simulink model "bicycle_kin_planCont"  (R2020b)
settings: Solver=FixedStepAuto  StartTime=0.0  StopTime=inf  FixedStep=0.02  RelTol=1e-3
model workspace (MAT data in the model file):
  SL_ROS_VariableLengthArrays_MaxSizes.CommonInfo.ArrayTruncateAction = 'EmitWarning'
  SL_ROS_VariableLengthArrays_MaxSizes.MsgTypeMap = containers.Map
  SL_ROS_VariableLengthArrays_MaxSizes.MsgTypeMap.serialization.keys = {'nav_msgs/Path'}
  SL_ROS_VariableLengthArrays_MaxSizes.MsgTypeMap.serialization.values{1}.PropertyName = 'Poses'
  SL_ROS_VariableLengthArrays_MaxSizes.MsgTypeMap.serialization.values{1}.DataType = 'geometry_msgs/PoseStamped'
  SL_ROS_VariableLengthArrays_MaxSizes.MsgTypeMap.serialization.values{1}.MaxLength = 25
  SL_ROS_VariableLengthArrays_MaxSizes.MsgTypeMap.serialization.uniformity = 0
  SL_ROS_VariableLengthArrays_MaxSizes.MsgTypeMap.serialization.keyType = 'char'
  SL_ROS_VariableLengthArrays_MaxSizes.MsgTypeMap.serialization.valueType = 'any'
undefined symbols (not defined in the file or in its folder): Angular, Linear
libraries: robotlib x12
settings Model: Creator=bascetta  LastModifiedBy=root
settings OptimizationCC: EnhancedBackFolding=on  PassReuseOutputArgsAs=Individual arguments  ZeroExternalMemoryAtStartup=off  ZeroInternalMemoryAtStartup=off  MaxStackSize=64  OptimizeBlockOrder=speed  DifferentSizesBufferReuse=on  OptimizationCustomize=off  EfficientTunableParamExpr=on
settings DebuggingCC: ParameterTunabilityLossMsg=error
settings HardwareCC: ProdBitPerPointer=32  ProdBitPerSizeT=32  ProdBitPerPtrDiffT=32  ProdLargestAtomicFloat=None  ProdIntDivRoundTo=Undefined  ProdEndianess=Unspecified  ProdWordSize=32  ProdHWDeviceType=Generic->Unspecified (assume 32-bit Generic)
settings SFSimCC: MATLABDynamicMemAlloc=off  SimTargetLang=C++
settings RTWCC: Description=Embedded Coder  SystemTargetFile=ert.tlc  HardwareBoard=Robot Operating System (ROS)  TLCOptions="-aInlineSetEventsForThisBaseRateFcn=TLC_FALSE -aSuppressMultiTaskScheduler=TLC_FALSE  -aRateBasedStepFcn=0"  GenCodeOnly=on  TemplateMakefile=ert_default_tmf  Toolchain=Catkin  TargetLang=C++
settings CodeAppCC: ForceParamTrailComments=on  IgnoreCustomStorageClasses=off  OperatorAnnotations=on  SimulinkDataObjDesc=on  SFDataObjDesc=on  InsertBlockDesc=on
settings ERTTargetCC: SupportVariableSizeSignals=on  ERTCustomFileTemplate=rostime_codertarget_file_process.tlc

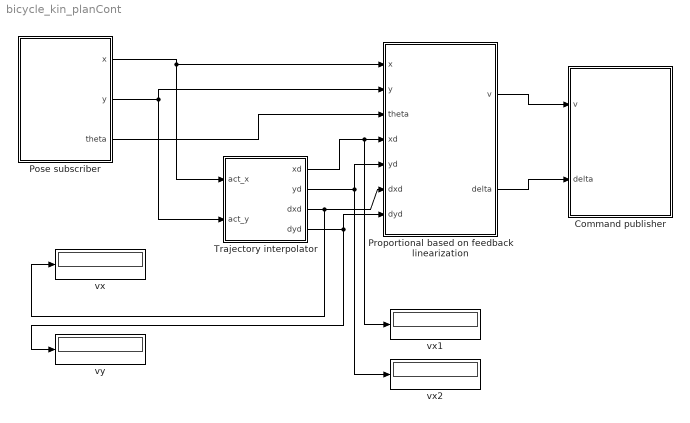
== system bicycle_kin_planCont ==
  Command publisher : Subsystem  mask{simPublishRate=50}
      mask prompts: simPublishRate "Publising rate [Hz]"
  Pose subscriber : Subsystem
  Proportional based on feedback linearization : Subsystem  mask{KP=0.5, Epsilon=0.5}
      mask prompts: KP "Proportional gain"; Epsilon "Distance of the point"
      mask TypeOptions Epsilon: point distance/Value
  Trajectory interpolator : Subsystem  mask{R=2.0}
      mask prompts: R "Ball radius to switch from one point to another"
  vx : Display
  vx1 : Display
  vx2 : Display
  vy : Display
  wires:
  Proportional based on feedback linearization/1(v) -> Command publisher/1(v)
  Proportional based on feedback linearization/2(delta) -> Command publisher/2(delta)
  Pose subscriber/1(x) -> Trajectory interpolator/1(act_x), Proportional based on feedback linearization/1(x)
  Pose subscriber/2(y) -> Trajectory interpolator/2(act_y), Proportional based on feedback linearization/2(y)
  Pose subscriber/3(theta) -> Proportional based on feedback linearization/3(theta)
  Trajectory interpolator/1(xd) -> Proportional based on feedback linearization/4(xd), vx1/1
  Trajectory interpolator/2(yd) -> vx2/1, Proportional based on feedback linearization/5(yd)
  Trajectory interpolator/3(dxd) -> vx/1, Proportional based on feedback linearization/6(dxd)
  Trajectory interpolator/4(dyd) -> vy/1, Proportional based on feedback linearization/7(dyd)

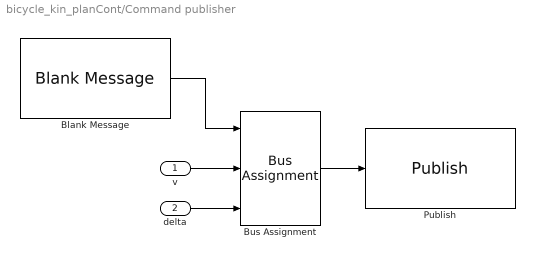
== system bicycle_kin_planCont/Command publisher ==
  v : Inport  SampleTime=1/simPublishRate
  delta : Inport  Port=2  SampleTime=1/simPublishRate
  Blank Message : robotlib/Blank Message  messageClass=Message  entityType=geometry_msgs/Twist  messageType=geometry_msgs/Twist  SampleTime=1/simPublishRate  legacyBusStruct=off
  Bus Assignment : BusAssignment  AssignedSignals=Linear.X,Angular.Z
  Publish : robotlib/Publish  topicSource=Specify your own  topic=/cmd_vel  messageType=geometry_msgs/Twist  legacyBusStruct=off  messageQueueLength=1
  wires:
  Bus Assignment/1 -> Publish/1
  Blank Message/1 -> Bus Assignment/1
  v/1 -> Bus Assignment/2
  delta/1 -> Bus Assignment/3

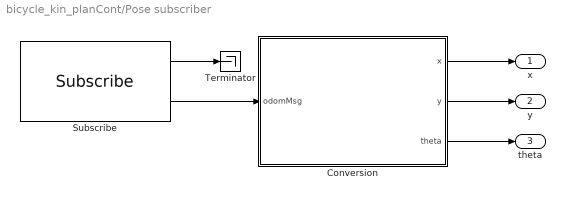
== system bicycle_kin_planCont/Pose subscriber ==
  Conversion : MATLAB Function  TreatAsAtomicUnit=on
  Subscribe : robotlib/Subscribe  topicSource=Specify your own  topic=/odom  messageType=nav_msgs/Odometry  SampleTime=-1  legacyBusStruct=off  messageQueueLength=1
  Terminator : Terminator
  x : Outport
  y : Outport  Port=2
  theta : Outport  Port=3
  wires:
  Subscribe/1 -> Terminator/1
  Subscribe/2 -> Conversion/1(odomMsg)
  Conversion/1(x) -> x/1
  Conversion/2(y) -> y/1
  Conversion/3(theta) -> theta/1

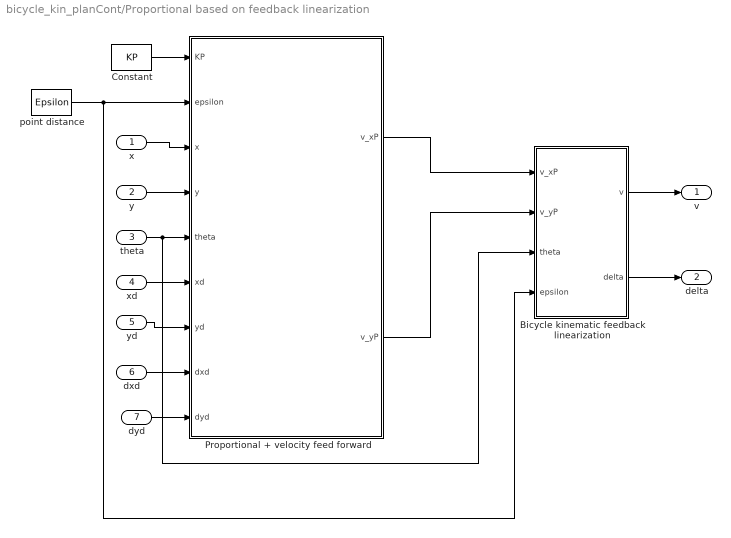
== system bicycle_kin_planCont/Proportional based on feedback linearization ==
  x : Inport
  y : Inport  Port=2
  theta : Inport  Port=3
  xd : Inport  Port=4
  yd : Inport  Port=5
  dxd : Inport  Port=6
  dyd : Inport  Port=7
  Bicycle kinematic feedback linearization : Subsystem  mask{CFD=1.1, RCD=1.6}
      mask prompts: CFD "Centre to Front distance"; RCD "Rear to Centre distance"
      mask TypeOptions CFD: Centre-Front Distance/Value
      mask TypeOptions RCD: Rear-Centre Distance/Value
  Constant : Constant  Value=KP
  Proportional + velocity feed forward : MATLAB Function  TreatAsAtomicUnit=on
  point distance : Constant  Value=Epsilon
  v : Outport  VectorParamsAs1DForOutWhenUnconnected=off
  delta : Outport  Port=2  VectorParamsAs1DForOutWhenUnconnected=off
  wires:
  Constant/1 -> Proportional + velocity feed forward/1(KP)
  x/1 -> Proportional + velocity feed forward/3(x)
  y/1 -> Proportional + velocity feed forward/4(y)
  xd/1 -> Proportional + velocity feed forward/6(xd)
  yd/1 -> Proportional + velocity feed forward/7(yd)
  Proportional + velocity feed forward/2(v_yP) -> Bicycle kinematic feedback linearization/2(v_yP)
  Proportional + velocity feed forward/1(v_xP) -> Bicycle kinematic feedback linearization/1(v_xP)
  Bicycle kinematic feedback linearization/2(delta) -> delta/1
  Bicycle kinematic feedback linearization/1(v) -> v/1
  point distance/1 -> Bicycle kinematic feedback linearization/4(epsilon), Proportional + velocity feed forward/2(epsilon)
  theta/1 -> Bicycle kinematic feedback linearization/3(theta), Proportional + velocity feed forward/5(theta)
  dxd/1 -> Proportional + velocity feed forward/8(dxd)
  dyd/1 -> Proportional + velocity feed forward/9(dyd)

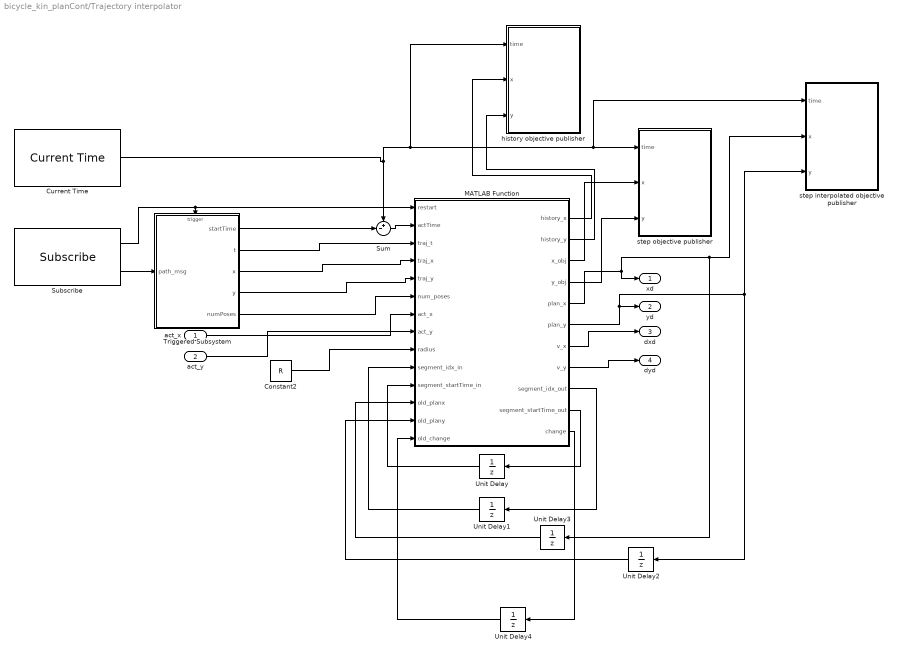
== system bicycle_kin_planCont/Trajectory interpolator ==
  act_x : Inport
  act_y : Inport  Port=2
  Constant2 : Constant  Value=R
  Current Time : robotlib/Current Time  OutputFormat=double  SampleTime=-1  ModelName=bicycle_kin_planCont
      settings: SourceProductBaseCode=RR
  MATLAB Function : MATLAB Function  TreatAsAtomicUnit=on
  Subscribe : robotlib/Subscribe  topicSource=Specify your own  topic=/plan  messageType=nav_msgs/Path  SampleTime=-1  legacyBusStruct=off  messageQueueLength=1
  Sum : Sum  Inputs=+-|
  Triggered Subsystem : Subsystem  TreatAsAtomicUnit=on
  Unit Delay{,1..4} (5 alike) : UnitDelay  SampleTime=-1  HasFrameUpgradeWarning=on
  history objective publisher : Subsystem  mask{simPublishRate=50}
      mask prompts: simPublishRate "Publising rate [Hz]"
  step interpolated objective publisher : Subsystem  mask{simPublishRate=50}
      mask prompts: simPublishRate "Publising rate [Hz]"
  step objective publisher : Subsystem  mask{simPublishRate=50}
      mask prompts: simPublishRate "Publising rate [Hz]"
  xd : Outport
  yd : Outport  Port=2
  dxd : Outport  Port=3
  dyd : Outport  Port=4
  wires:
  MATLAB Function/9(segment_idx_out) -> Unit Delay1/1
  act_x/1 -> MATLAB Function/7(act_x)
  Unit Delay1/1 -> MATLAB Function/10(segment_idx_in)
  MATLAB Function/6(plan_y) -> Unit Delay2/1, step interpolated objective publisher/3(y), yd/1
  Unit Delay/1 -> MATLAB Function/11(segment_startTime_in)
  Current Time/1 -> Sum/1, history objective publisher/1(time), step interpolated objective publisher/1(time), step objective publisher/1(time)
  Triggered Subsystem/4(y) -> MATLAB Function/5(traj_y)
  Subscribe/2 -> Triggered Subsystem/1(path_msg)
  Triggered Subsystem/2(t) -> MATLAB Function/3(traj_t)
  Constant2/1 -> MATLAB Function/9(radius)
  MATLAB Function/10(segment_startTime_out) -> Unit Delay/1
  Triggered Subsystem/1(startTime) -> Sum/2
  act_y/1 -> MATLAB Function/8(act_y)
  MATLAB Function/5(plan_x) -> Unit Delay3/1, step interpolated objective publisher/2(x), xd/1
  Sum/1 -> MATLAB Function/2(actTime)
  Triggered Subsystem/5(numPoses) -> MATLAB Function/6(num_poses)
  Subscribe/1 -> Triggered Subsystem/Trigger, MATLAB Function/1(restart)
  MATLAB Function/7(v_x) -> dxd/1
  MATLAB Function/8(v_y) -> dyd/1
  MATLAB Function/3(x_obj) -> step objective publisher/2(x)
  MATLAB Function/4(y_obj) -> step objective publisher/3(y)
  Unit Delay3/1 -> MATLAB Function/12(old_planx)
  Unit Delay2/1 -> MATLAB Function/13(old_plany)
  MATLAB Function/1(history_x) -> history objective publisher/2(x)
  MATLAB Function/2(history_y) -> history objective publisher/3(y)
  Triggered Subsystem/3(x) -> MATLAB Function/4(traj_x)
  MATLAB Function/11(change) -> Unit Delay4/1
  Unit Delay4/1 -> MATLAB Function/14(old_change)

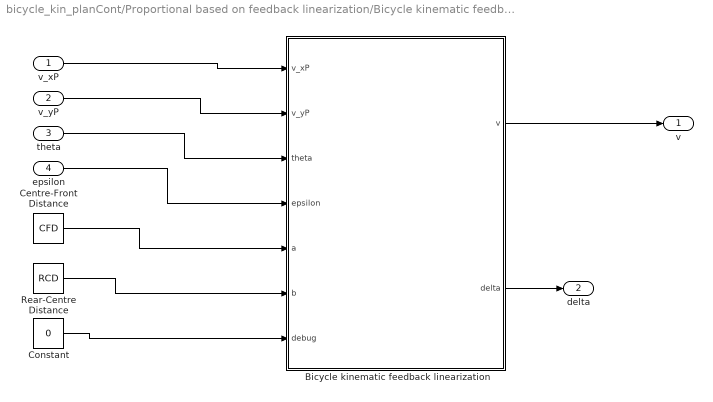
== system bicycle_kin_planCont/Proportional based on feedback linearization/Bicycle kinematic feedback linearization ==
  v_xP : Inport
  v_yP : Inport  Port=2
  theta : Inport  Port=3
  epsilon : Inport  Port=4
  Bicycle kinematic feedback linearization : MATLAB Function  TreatAsAtomicUnit=on
  Centre-Front Distance : Constant  Value=CFD
  Constant : Constant  Value=0
  Rear-Centre Distance : Constant  Value=RCD
  v : Outport  VectorParamsAs1DForOutWhenUnconnected=off
  delta : Outport  Port=2  VectorParamsAs1DForOutWhenUnconnected=off
  wires:
  Bicycle kinematic feedback linearization/2(delta) -> delta/1
  v_yP/1 -> Bicycle kinematic feedback linearization/2(v_yP)
  Bicycle kinematic feedback linearization/1(v) -> v/1
  v_xP/1 -> Bicycle kinematic feedback linearization/1(v_xP)
  theta/1 -> Bicycle kinematic feedback linearization/3(theta)
  epsilon/1 -> Bicycle kinematic feedback linearization/4(epsilon)
  Centre-Front Distance/1 -> Bicycle kinematic feedback linearization/5(a)
  Rear-Centre Distance/1 -> Bicycle kinematic feedback linearization/6(b)
  Constant/1 -> Bicycle kinematic feedback linearization/7(debug)

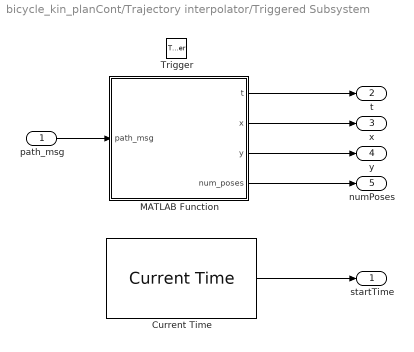
== system bicycle_kin_planCont/Trajectory interpolator/Triggered Subsystem ==
  path_msg : Inport
  Trigger : TriggerPort  VariantControl=Variant
  Current Time : robotlib/Current Time  OutputFormat=double  SampleTime=-1  ModelName=bicycle_kin_planCont
      settings: SourceProductBaseCode=RR
  MATLAB Function : MATLAB Function  TreatAsAtomicUnit=on
  startTime : Outport
  t : Outport  Port=2
  x : Outport  Port=3
  y : Outport  Port=4
  numPoses : Outport  Port=5
  wires:
  path_msg/1 -> MATLAB Function/1(path_msg)
  Current Time/1 -> startTime/1
  MATLAB Function/1(t) -> t/1
  MATLAB Function/3(y) -> y/1
  MATLAB Function/2(x) -> x/1
  MATLAB Function/4(num_poses) -> numPoses/1

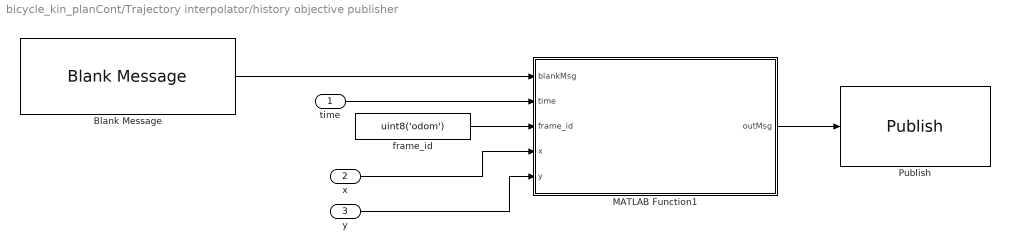
== system bicycle_kin_planCont/Trajectory interpolator/history objective publisher ==
  time : Inport  SampleTime=1/simPublishRate
  x : Inport  Port=2  SampleTime=1/simPublishRate
  y : Inport  Port=3  SampleTime=1/simPublishRate
  Blank Message : robotlib/Blank Message  messageClass=Message  entityType=geometry_msgs/PointStamped  messageType=geometry_msgs/PointStamped  SampleTime=inf  legacyBusStruct=off
  MATLAB Function1 : MATLAB Function  TreatAsAtomicUnit=on
  Publish : robotlib/Publish  topicSource=Specify your own  topic=/last_objective  messageType=geometry_msgs/PointStamped  legacyBusStruct=off  messageQueueLength=1
  frame_id : Constant  Value=uint8('odom')
  wires:
  time/1 -> MATLAB Function1/2(time)
  x/1 -> MATLAB Function1/4(x)
  y/1 -> MATLAB Function1/5(y)
  MATLAB Function1/1(outMsg) -> Publish/1
  Blank Message/1 -> MATLAB Function1/1(blankMsg)
  frame_id/1 -> MATLAB Function1/3(frame_id)

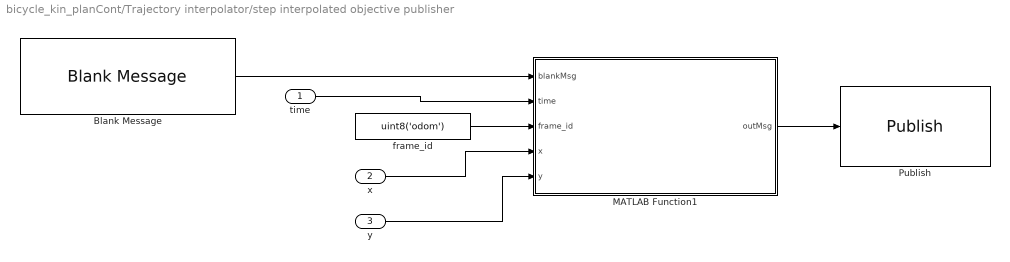
== system bicycle_kin_planCont/Trajectory interpolator/step interpolated objective publisher ==
  time : Inport  SampleTime=1/simPublishRate
  x : Inport  Port=2  SampleTime=1/simPublishRate
  y : Inport  Port=3  SampleTime=1/simPublishRate
  Blank Message : robotlib/Blank Message  messageClass=Message  entityType=geometry_msgs/PointStamped  messageType=geometry_msgs/PointStamped  SampleTime=inf  legacyBusStruct=off
  MATLAB Function1 : MATLAB Function  TreatAsAtomicUnit=on
  Publish : robotlib/Publish  topicSource=Specify your own  topic=/inter_objective  messageType=geometry_msgs/PointStamped  legacyBusStruct=off  messageQueueLength=1
  frame_id : Constant  Value=uint8('odom')
  wires:
  time/1 -> MATLAB Function1/2(time)
  x/1 -> MATLAB Function1/4(x)
  y/1 -> MATLAB Function1/5(y)
  MATLAB Function1/1(outMsg) -> Publish/1
  Blank Message/1 -> MATLAB Function1/1(blankMsg)
  frame_id/1 -> MATLAB Function1/3(frame_id)

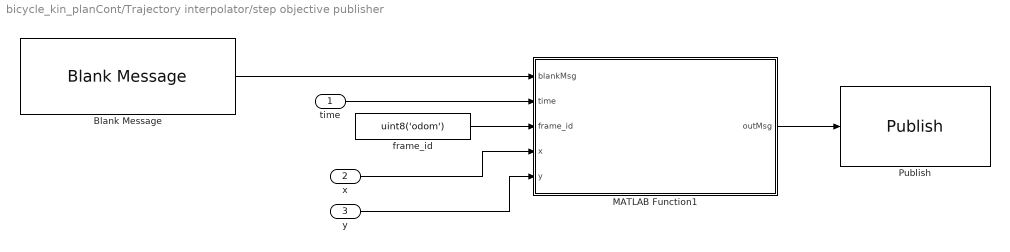
== system bicycle_kin_planCont/Trajectory interpolator/step objective publisher ==
  time : Inport  SampleTime=1/simPublishRate
  x : Inport  Port=2  SampleTime=1/simPublishRate
  y : Inport  Port=3  SampleTime=1/simPublishRate
  Blank Message : robotlib/Blank Message  messageClass=Message  entityType=geometry_msgs/PointStamped  messageType=geometry_msgs/PointStamped  SampleTime=inf  legacyBusStruct=off
  MATLAB Function1 : MATLAB Function  TreatAsAtomicUnit=on
  Publish : robotlib/Publish  topicSource=Specify your own  topic=/objective  messageType=geometry_msgs/PointStamped  legacyBusStruct=off  messageQueueLength=1
  frame_id : Constant  Value=uint8('odom')
  wires:
  time/1 -> MATLAB Function1/2(time)
  x/1 -> MATLAB Function1/4(x)
  y/1 -> MATLAB Function1/5(y)
  MATLAB Function1/1(outMsg) -> Publish/1
  Blank Message/1 -> MATLAB Function1/1(blankMsg)
  frame_id/1 -> MATLAB Function1/3(frame_id)

== matlab function bicycle_kin_planCont/Trajectory interpolator/Triggered Subsystem/MATLAB Function ==
  data: t output; path_msg input; x output; y output; num_poses output
function [t,x,y,num_poses]  = pathMsg2traj(path_msg)

t = zeros(1,length(path_msg.Poses));
x = zeros(1,length(path_msg.Poses));
y = zeros(1,length(path_msg.Poses));
for k=1:length(path_msg.Poses)
    t(k) = path_msg.Poses(k).Header.Stamp.Sec+path_msg.Poses(k).Header.Stamp.Nsec*1e-9;
    x(k) = path_msg.Poses(k).Pose.Position.X;
    y(k) = path_msg.Poses(k).Pose.Position.Y;
end

num_poses = path_msg.Poses_SL_Info.ReceivedLength;

== matlab function bicycle_kin_planCont/Trajectory interpolator/step objective publisher/MATLAB Function1 ==
  data: blankMsg input; outMsg output Bus: SL_Bus_bicycle_kin_planCont_geometry_msgs_PointStamped; time input; frame_id input; x input; y input
function outMsg = currentObjectivePublisher(blankMsg,time,frame_id,x,y)
% Writing the message header
blankMsg.Header.Stamp.Sec = fix(time);
blankMsg.Header.Stamp.Nsec = fix((time-fix(time))*1e9);
blankMsg.Header.FrameId(1:length(frame_id)) = frame_id;
blankMsg.Header.FrameId_SL_Info.CurrentLength = uint32(length(frame_id));

% Writing position
blankMsg.Point.X = x;
blankMsg.Point.Y = y;
blankMsg.Point.Z = 0;

outMsg = blankMsg;

== matlab function bicycle_kin_planCont/Trajectory interpolator/history objective publisher/MATLAB Function1 ==
  data: blankMsg input; outMsg output Bus: SL_Bus_bicycle_kin_planCont_geometry_msgs_PointStamped; time input; frame_id input; x input; y input
function outMsg = currentObjectivePublisher(blankMsg,time,frame_id,x,y)
% Writing the message header
blankMsg.Header.Stamp.Sec = fix(time);
blankMsg.Header.Stamp.Nsec = fix((time-fix(time))*1e9);
blankMsg.Header.FrameId(1:length(frame_id)) = frame_id;
blankMsg.Header.FrameId_SL_Info.CurrentLength = uint32(length(frame_id));

% Writing position
blankMsg.Point.X = x;
blankMsg.Point.Y = y;
blankMsg.Point.Z = 0;

outMsg = blankMsg;

== matlab function bicycle_kin_planCont/Trajectory interpolator/step interpolated objective publisher/MATLAB Function1 ==
  data: blankMsg input; outMsg output Bus: SL_Bus_bicycle_kin_planCont_geometry_msgs_PointStamped; time input; frame_id input; x input; y input
function outMsg = currentObjectivePublisher(blankMsg,time,frame_id,x,y)
% Writing the message header
blankMsg.Header.Stamp.Sec = fix(time);
blankMsg.Header.Stamp.Nsec = fix((time-fix(time))*1e9);
blankMsg.Header.FrameId(1:length(frame_id)) = frame_id;
blankMsg.Header.FrameId_SL_Info.CurrentLength = uint32(length(frame_id));

% Writing position
blankMsg.Point.X = x;
blankMsg.Point.Y = y;
blankMsg.Point.Z = 0;

outMsg = blankMsg;

== matlab function bicycle_kin_planCont/Proportional based on feedback linearization/Bicycle kinematic feedback linearization/Bicycle kinematic feedback linearization ==
  data: v_xP input; v output; v_yP input; delta output; theta input; epsilon input; a input; b input; debug input
function [v,delta] = fblin_bicycle_kinematic(v_xP,v_yP,theta,epsilon, a, b, debug)

l = a + b;

v = v_xP*cos(theta)+v_yP*sin(theta);

num = v_yP*cos(theta)-v_xP*sin(theta);
den = v_xP*cos(theta)+v_yP*sin(theta);

if (num == 0 && den == 0)
    delta = 0;
else    
    delta = atan((l/epsilon)*(num)/(den));
end
    
%limiting steer angle to 45 degrees
if(delta > 0.7) 
    delta = 0.7;
elseif (delta < -0.7)
    delta = -0.7;
end

if(debug == 1)
    delta = 0;
    v = 0;
end

== matlab function bicycle_kin_planCont/Trajectory interpolator/MATLAB Function ==
  data: history_x output; history_y output; x_obj output; y_obj output; restart input; plan_x output; plan_y output; v_x output; v_y output; actTime input; traj_t input; traj_x input; traj_y input; num_poses input; act_x input; act_y input; radius input; segment_idx_in input; segment_startTime_in input; segment_idx_out output; segment_startTime_out output; old_planx input; old_plany input; change output; old_change input
function [history_x,history_y,x_obj,y_obj, plan_x,plan_y,v_x,v_y,segment_idx_out,segment_startTime_out,change] = interpolator(restart,actTime,traj_t,traj_x,traj_y,num_poses,act_x,act_y,radius,segment_idx_in,segment_startTime_in, old_planx, old_plany, old_change)

% Initialize input/output variables
segment_idx_out = segment_idx_in;
segment_startTime_out = segment_startTime_in;
change = 0;
jump = 0;

% Start and restart logic
if (segment_idx_in==0) && (restart==0)
    plan_x = act_x;
    plan_y = act_y;
    x_obj = act_x;
    y_obj = act_y;
    history_x = act_x;
    history_y = act_y;
    segment_idx_out = 0;
    v_x=0;
    v_y=0;
    return;
end

if (restart==1)
    segment_idx_out = 2;
    segment_startTime_out = actTime;
    plan_x = traj_x(segment_idx_out);
    plan_y = traj_y(segment_idx_out);
    jump = 1;
end

% Time for trajectory interpolation
t = actTime-segment_startTime_in;

x_obj = traj_x(segment_idx_out+1);
y_obj = traj_y(segment_idx_out+1);
history_x = traj_x(segment_idx_out);
history_y = traj_y(segment_idx_out);


% Compute the planned point interpolating between P(idx) and P(idx+1)
if (segment_idx_out>=num_poses)
    % No more interpolated point needed
    plan_x = traj_x(num_poses);
    plan_y = traj_y(num_poses);
    v_x=0;
    v_y=0;
else
    v_x = (traj_x(segment_idx_out+1)-traj_x(segment_idx_out))/(traj_t(segment_idx_out+1)-traj_t(segment_idx_out));
    v_y = (traj_y(segment_idx_out+1)-traj_y(segment_idx_out))/(traj_t(segment_idx_out+1)-traj_t(segment_idx_out));
    
	if(traj_x(segment_idx_out+1)-traj_x(segment_idx_out) ~= 0)
		m = (traj_y(segment_idx_out+1)-traj_y(segment_idx_out))/(traj_x(segment_idx_out+1)-traj_x(segment_idx_out));
		q = traj_y(segment_idx_out);
   
		if (sqrt((act_x-old_planx)^2+(act_y-old_plany)^2)<=(radius/1.5))
			if(jump == 1)
				jump = 0;
				plan_x = old_planx;
				plan_y = old_plany;
			else
				if(old_change == 1)
					change = 0;
					if(traj_x(segment_idx_out+1)>traj_x(segment_idx_out))
						plan_x = traj_x(segment_idx_out) + 1;
					else
						plan_x = traj_x(segment_idx_out) - 1;
					end
					plan_y = m*(plan_x-traj_x(segment_idx_out)) + q;
				else
					if(traj_x(segment_idx_out+1)>traj_x(segment_idx_out))
						plan_x = old_planx + 1;
					else
						plan_x = old_planx - 1;
					end
					plan_y = m*(plan_x-traj_x(segment_idx_out)) +q;
				end
			end
		else
			plan_x = old_planx;
			plan_y = old_plany;
		end
	else %case vertical line
		if (sqrt((act_x-old_planx)^2+(act_y-old_plany)^2)<=(radius/1.5))
			if(jump == 1)
				jump = 0;
				plan_x = old_planx;
				plan_y = old_plany;
			else
				if(old_change == 1)
					change = 0;
					if(traj_y(segment_idx_out+1)>traj_y(segment_idx_out))
						plan_y = traj_y(segment_idx_out) + 1;
					else
						plan_y = traj_y(segment_idx_out) - 1;
					end
					plan_x = old_planx;
				else
					if(traj_y(segment_idx_out+1)>traj_y(segment_idx_out))
						plan_y = old_plany + 1;
					else
						plan_y = old_plany - 1;
					end
					plan_x = old_planx;
				end
			end
		else
			plan_x = old_planx;
			plan_y = old_plany;
		end
	
	end
    
end


% Update the index idx
if (segment_idx_out<num_poses)
    if (sqrt((act_x-traj_x(segment_idx_out+1))^2+(act_y-traj_y(segment_idx_out+1))^2)<=radius)
        
        segment_idx_out = segment_idx_out+1;
        if(traj_x(segment_idx_out+1)-traj_x(segment_idx_out) ~= 0)
			m = (traj_y(segment_idx_out+1)-traj_y(segment_idx_out))/(traj_x(segment_idx_out+1)-traj_x(segment_idx_out));
			q = traj_y(segment_idx_out);
			if(traj_x(segment_idx_out+1)>traj_x(segment_idx_out))
				xi = traj_x(segment_idx_out) + 0.5;
			else
				xi = traj_x(segment_idx_out) - 0.5;
			end
			yi = m*(xi - traj_x(segment_idx_out))  + q;
        else %case vertical line
			if(traj_y(segment_idx_out+1)>traj_y(segment_idx_out))
				yi = traj_y(segment_idx_out) + 0.5;
			else
				yi = traj_y(segment_idx_out) - 0.5;
			end
			xi = traj_x(segment_idx_out);
		end
		
		
        dist_x = (xi - act_x)/2;
        x_half = (act_x + dist_x);
		dist_y = (yi - act_y)/2;
        y_half = (act_y + dist_y);
        
        plan_x = x_half;
        plan_y = y_half;
        
        change = 1;
        segment_startTime_out = actTime;
    end
end

== matlab function bicycle_kin_planCont/Proportional based on feedback linearization/Proportional + velocity feed forward ==
  data: KP input; epsilon input; x input; v_xP output; y input; theta input; xd input; yd input; v_yP output; dxd input; dyd input
function [v_xP,v_yP] = Proportional_VelocityFF(KP,epsilon,x,y,theta,xd,yd,dxd,dyd)

% Point P transformation (position)
xP = x+epsilon*cos(theta);
yP = y+epsilon*sin(theta);

xPd = xd+epsilon*cos(theta);
yPd = yd+epsilon*sin(theta);

% Control law
v_xP = dxd + KP*(xPd-xP);
v_yP = dyd + KP*(yPd-yP);

== matlab function bicycle_kin_planCont/Pose subscriber/Conversion ==
  data: x output; odomMsg input; y output; theta output
function [x,y,theta]  = odom_2_xytheta(odomMsg)

% Position
x = odomMsg.Pose.Pose.Position.X;
y = odomMsg.Pose.Pose.Position.Y;

% Orientation
orientation = [odomMsg.Pose.Pose.Orientation.X,odomMsg.Pose.Pose.Orientation.Y,...
    odomMsg.Pose.Pose.Orientation.Z,odomMsg.Pose.Pose.Orientation.W];

if all(orientation==zeros(1,4))
    theta = 0;
else
    eul = quat2eul(orientation,'ZYX');
    theta = eul(3);
end
